simulink model "Chinh_Luu"  (R2019a)
settings: Solver=VariableStepAuto  StartTime=0.0  StopTime=0.5  RelTol=1e-3
libraries: powerlib x23, powerlib_meascontrol x6
settings Model: Creator=Admin  LastModifiedBy=Admin

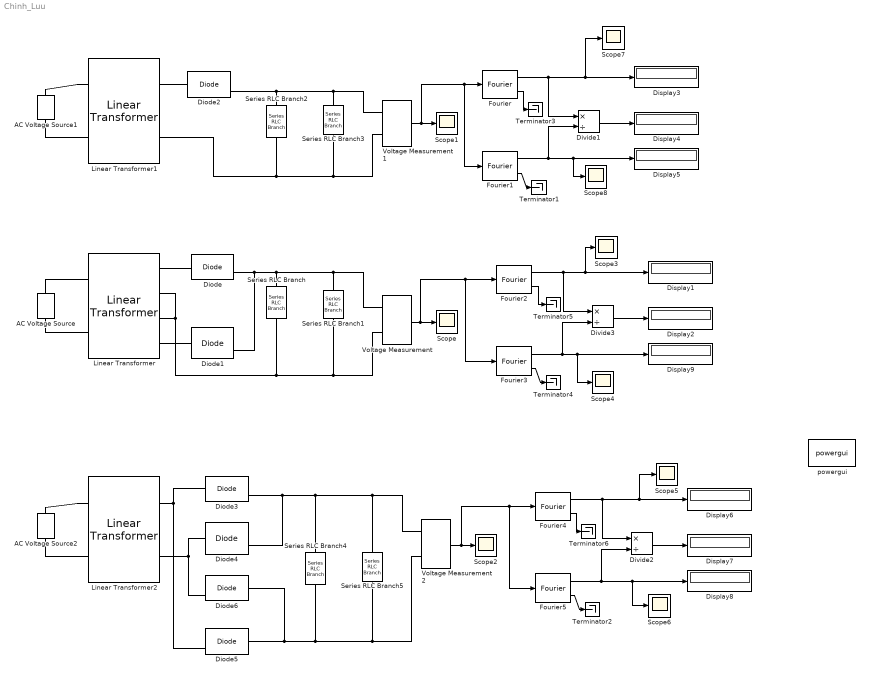
== system Chinh_Luu ==
  AC Voltage Source : powerlib/Electrical Sources/AC Voltage Source  Amplitude=120*sqrt(2)  Phase=0  Frequency=50  SampleTime=0  Measurements=None  BusType=swing  Pref=10e3  Qref=0  Qmin=-inf  Qmax=+inf
      settings: SourceProductName=Simscape Electrical
  AC Voltage Source1 : powerlib/Electrical Sources/AC Voltage Source  Amplitude=100*sqrt(2)  Phase=0  Frequency=50  SampleTime=0  Measurements=None  BusType=swing  Pref=10e3  Qref=0  Qmin=-inf  Qmax=+inf
      settings: SourceProductName=Simscape Electrical
  AC Voltage Source2 : powerlib/Electrical Sources/AC Voltage Source  Amplitude=100*sqrt(2)  Phase=0  Frequency=50  SampleTime=0  Measurements=None  BusType=swing  Pref=10e3  Qref=0  Qmin=-inf  Qmax=+inf
      settings: SourceProductName=Simscape Electrical
  Diode{,1..6} (7 alike) : powerlib/Power Electronics/Diode  Ron=0.001  Lon=0  Vf=0.8  IC=0  UseSnubber=0  Rs=500  Cs=250e-9  Measurements=on
      settings: SourceProductName=Simscape Electrical
  Display{1..9} (9 alike) : Display
  Divide1 : Product  Inputs=*/
  Divide2 : Product  Inputs=*/
  Divide3 : Product  Inputs=*/
  Fourier : powerlib_meascontrol/Measurements/Fourier  Freq=50  n=1  InInit=[0, 0]  Ts=0
      settings: SourceProductName=Simscape Electrical
  Fourier1 : powerlib_meascontrol/Measurements/Fourier  Freq=50  n=0  InInit=[0, 0]  Ts=0
      settings: SourceProductName=Simscape Electrical
  Fourier2 : powerlib_meascontrol/Measurements/Fourier  Freq=100  n=1  InInit=[0, 0]  Ts=0
      settings: SourceProductName=Simscape Electrical
  Fourier3 : powerlib_meascontrol/Measurements/Fourier  Freq=100  n=0  InInit=[0, 0]  Ts=0
      settings: SourceProductName=Simscape Electrical
  Fourier4 : powerlib_meascontrol/Measurements/Fourier  Freq=100  n=1  InInit=[0, 0]  Ts=0
      settings: SourceProductName=Simscape Electrical
  Fourier5 : powerlib_meascontrol/Measurements/Fourier  Freq=100  n=0  InInit=[0, 0]  Ts=0
      settings: SourceProductName=Simscape Electrical
  Linear Transformer : powerlib/Elements/Linear Transformer  UNITS=SI  NominalPower=[ 60 50 ]  winding1=[120 0 0]  winding2=[20 0.03 0.02]  ThreeWindings=on  winding3=[20 0.03 0.02]  RmLm=[Inf Inf]  Measurements=None  DataType=on
      settings: SourceProductName=Simscape Electrical
  Linear Transformer1 : powerlib/Elements/Linear Transformer  UNITS=SI  NominalPower=[60 50 ]  winding1=[100 0 0]  winding2=[15 0.03 0.02]  ThreeWindings=off  winding3=[3.15e+05 3.3075e+06 4.2112e+05]  RmLm=[Inf Inf]  Measurements=None  DataType=on
      settings: SourceProductName=Simscape Electrical
  Linear Transformer2 : powerlib/Elements/Linear Transformer  UNITS=SI  NominalPower=[60 50 ]  winding1=[100 0 0]  winding2=[15 0.03 0.02]  ThreeWindings=off  winding3=[3.15e+05 3.3075e+06 4.2112e+05]  RmLm=[Inf Inf]  Measurements=None  DataType=on
      settings: SourceProductName=Simscape Electrical
  Scope{,1..8} (9 alike) : Scope
  Series RLC Branch : powerlib/Elements/Series RLC Branch  LConnTagsString=__new0  RConnTagsString=__new0  BranchType=C  Resistance=1  Inductance=1e-3  SetiL0=off  InitialCurrent=0  Capacitance=10000e-06  Setx0=off  InitialVoltage=0  Measurements=None
      settings: SourceProductName=Simscape Electrical
  Series RLC Branch1 : powerlib/Elements/Series RLC Branch  LConnTagsString=__new0  RConnTagsString=__new0  BranchType=R  Resistance=10  Inductance=1e-3  SetiL0=off  InitialCurrent=0  Capacitance=1e-6  Setx0=off  InitialVoltage=0  Measurements=None
      settings: SourceProductName=Simscape Electrical
  Series RLC Branch2 : powerlib/Elements/Series RLC Branch  LConnTagsString=__new0  RConnTagsString=__new0  BranchType=C  Resistance=1  Inductance=1e-3  SetiL0=off  InitialCurrent=0  Capacitance=20000e-06  Setx0=off  InitialVoltage=0  Measurements=None
      settings: SourceProductName=Simscape Electrical
  Series RLC Branch3 : powerlib/Elements/Series RLC Branch  LConnTagsString=__new0  RConnTagsString=__new0  BranchType=R  Resistance=5  Inductance=1e-3  SetiL0=off  InitialCurrent=0  Capacitance=1e-6  Setx0=off  InitialVoltage=0  Measurements=None
      settings: SourceProductName=Simscape Electrical
  Series RLC Branch4 : powerlib/Elements/Series RLC Branch  LConnTagsString=__new0  RConnTagsString=__new0  BranchType=C  Resistance=1  Inductance=1e-3  SetiL0=off  InitialCurrent=0  Capacitance=20000e-6  Setx0=off  InitialVoltage=0  Measurements=None
      settings: SourceProductName=Simscape Electrical
  Series RLC Branch5 : powerlib/Elements/Series RLC Branch  LConnTagsString=__new0  RConnTagsString=__new0  BranchType=R  Resistance=15  Inductance=1e-3  SetiL0=off  InitialCurrent=0  Capacitance=1e-6  Setx0=off  InitialVoltage=0  Measurements=None
      settings: SourceProductName=Simscape Electrical
  Terminator{1..6} (6 alike) : Terminator
  Voltage Measurement : powerlib/Measurements/Voltage Measurement  PhasorSimulation=off  OutputType=Magnitude  PSBequivalent=0
      settings: SourceProductName=Simscape Electrical
  Voltage Measurement1 : powerlib/Measurements/Voltage Measurement  PhasorSimulation=off  OutputType=Magnitude  PSBequivalent=0
      settings: SourceProductName=Simscape Electrical
  Voltage Measurement2 : powerlib/Measurements/Voltage Measurement  PhasorSimulation=off  OutputType=Complex  PSBequivalent=0
      settings: SourceProductName=Simscape Electrical
  powergui : powerlib/powergui  Priority=1  SimulationMode=Continuous  SampleTime=50e-6  frequency=60  Iterations=50  frequencyindice=50  Pbase=100e6  ErrMax=1e-4  UnitsV=kV  UnitsW=MW  buscounter=0  FunctionMessages=off  echomessages=off  EnableUseOfTLC=off  CurrentSourceSwitches=off  DisableSnubberDevices=off  DisableRonSwitches=off  DisableVfSwitches=off  DisplayEquations=off  AutomaticDiscreteSolvers=off  SolverType=Tustin/Backward Euler (TBE)  Interpol=off  ExternalGateDelay=off  methode=off  Ts=100  x0status=blocks  SPID=off  SwTol=0  HookPort=off  NonlinearTolerance=0  nMaxIteration=15  ContinueOnMaxIteration=off  RestoreLinks=warning  ResistiveCurrentMeasurement=off  Frange=[0:2:500]  Ylog=off  Xlog=on  ShowGrid=off  save=off  variable=ZData  structure=0  ZoomFFT=off  StartTime=0.0  cycles=1  DisplayStyle=1  fundamental=60  FreqAxis=off  MaxFrequency=1000  frequencyindicesteady=1  RmsSteady=1  display=off
      settings: SourceProductName=Simscape Electrical
  wires:
  Voltage Measurement/1 -> Fourier3/1, Fourier2/1, Scope/1
  Divide1/1 -> Display4/1
  Voltage Measurement1/1 -> Fourier1/1, Fourier/1, Scope1/1
  Voltage Measurement2/1 -> Fourier5/1, Fourier4/1, Scope2/1
  Fourier/2 -> Terminator3/1
  Fourier1/2 -> Terminator1/1
  Fourier/1 -> Divide1/1, Scope7/1, Display3/1
  Fourier1/1 -> Scope8/1, Display5/1, Divide1/2
  Fourier2/2 -> Terminator5/1
  Fourier3/1 -> Scope4/1, Display9/1, Divide3/2
  Fourier3/2 -> Terminator4/1
  Fourier2/1 -> Divide3/1, Scope3/1, Display1/1
  Divide3/1 -> Display2/1
  Fourier4/2 -> Terminator6/1
  Fourier5/1 -> Scope6/1, Display8/1, Divide2/2
  Fourier5/2 -> Terminator2/1
  Fourier4/1 -> Divide2/1, Display6/1, Scope5/1
  Divide2/1 -> Display7/1
  connections:
  Linear Transformer/RConn1 -- Diode/LConn1
  Diode/RConn1 -- Diode1/RConn1 -- Series RLC Branch1/LConn1 -- Voltage Measurement/LConn1 -- Series RLC Branch/LConn1
  Linear Transformer/RConn2 -- Series RLC Branch1/RConn1 -- Voltage Measurement/LConn2 -- Series RLC Branch/RConn1 -- Linear Transformer/RConn3
  Diode1/LConn1 -- Linear Transformer/RConn4
  Linear Transformer/LConn1 -- AC Voltage Source/RConn1
  Linear Transformer/LConn2 -- AC Voltage Source/LConn1
  Diode2/RConn1 -- Series RLC Branch2/LConn1 -- Series RLC Branch3/LConn1 -- Voltage Measurement1/LConn1
  Series RLC Branch2/RConn1 -- Series RLC Branch3/RConn1 -- Voltage Measurement1/LConn2 -- Linear Transformer1/RConn2
  Linear Transformer1/LConn2 -- AC Voltage Source1/LConn1
  Linear Transformer1/RConn1 -- Diode2/LConn1
  Linear Transformer1/LConn1 -- AC Voltage Source1/RConn1
  Series RLC Branch4/LConn1 -- Diode4/RConn1 -- Diode3/RConn1 -- Voltage Measurement2/LConn1 -- Series RLC Branch5/LConn1
  Series RLC Branch4/RConn1 -- Diode6/LConn1 -- Diode5/LConn1 -- Series RLC Branch5/RConn1 -- Voltage Measurement2/LConn2
  Linear Transformer2/LConn2 -- AC Voltage Source2/LConn1
  Linear Transformer2/LConn1 -- AC Voltage Source2/RConn1
  Diode6/RConn1 -- Linear Transformer2/RConn2 -- Diode4/LConn1
  Linear Transformer2/RConn1 -- Diode5/RConn1 -- Diode3/LConn1
